simulink model "cc"  (R2015b)
settings: Solver=VariableStepAuto  StartTime=0.0  StopTime=20  RelTol=1e-3
settings Model: Creator=Oscar  LastModifiedBy=Oscar
settings DebuggingCC: MaxConsecutiveZCsMsg=none

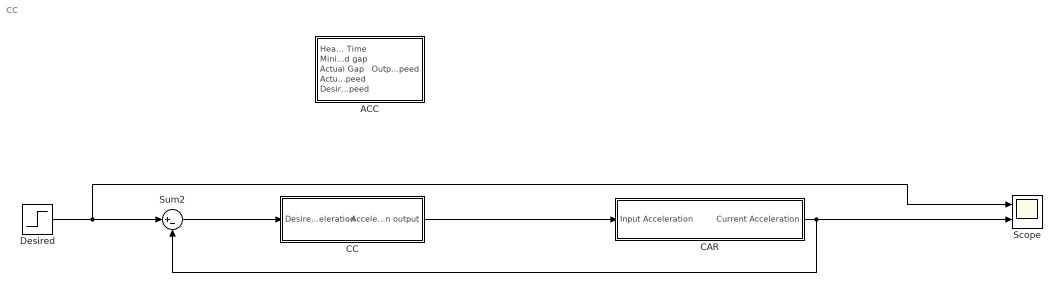
== system cc ==
  ACC : Subsystem
  "CAR " : Subsystem
  CC : Subsystem
  Desired : Step  After=1.3  SampleTime=0.0001
  Scope : Scope  NumInputPorts=2
  Sum2 : Sum  Inputs=|+-
  wires:
  Desired/1 -> Scope/1, Sum2/1
  "CAR "/1("Current Acceleration ") -> Sum2/2, Scope/2
  Sum2/1 -> CC/1(Desired Acceleration)
  CC/1(Acceleration output) -> "CAR "/1(Input Acceleration)

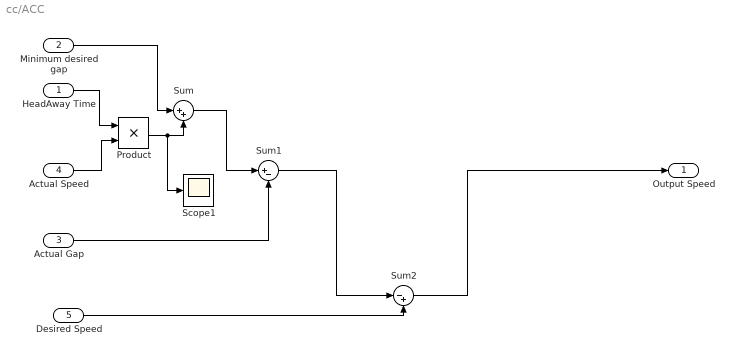
== system cc/ACC ==
  HeadAway Time : Inport
  Minimum desired gap : Inport  Port=2
  " Actual Gap" : Inport  Port=3
  " Actual Speed" : Inport  Port=4
  Desired Speed : Inport  Port=5
  Product : Product
  Scope1 : Scope
  Sum : Sum  Inputs=|++
  Sum1 : Sum  Inputs=|+-
  Sum2 : Sum  Inputs=|-+
  Output Speed : Outport
  wires:
  HeadAway Time/1 -> Product/1
  " Actual Speed"/1 -> Product/2
  Minimum desired gap/1 -> Sum/1
  Product/1 -> Scope1/1, Sum/2
  " Actual Gap"/1 -> Sum1/2
  Sum/1 -> Sum1/1
  Sum2/1 -> Output Speed/1
  Desired Speed/1 -> Sum2/2
  Sum1/1 -> Sum2/1

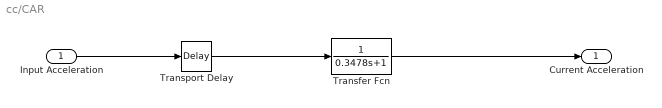
== system cc/CAR  ==
  Input Acceleration : Inport
  Transfer Fcn : TransferFcn  Denominator=[0.3478 1]
  Transport Delay : TransportDelay  DelayTime=0.4425
  "Current Acceleration " : Outport
  wires:
  Transfer Fcn/1 -> "Current Acceleration "/1
  Input Acceleration/1 -> Transport Delay/1
  Transport Delay/1 -> Transfer Fcn/1

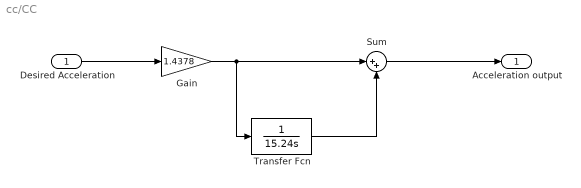
== system cc/CC ==
  Desired Acceleration : Inport
  Gain : Gain  Gain=1.4378
  Sum : Sum  Inputs=|++
  Transfer Fcn : TransferFcn  Denominator=[15.24 0]
  Acceleration output : Outport
  wires:
  Desired Acceleration/1 -> Gain/1
  Gain/1 -> Transfer Fcn/1, Sum/1
  Transfer Fcn/1 -> Sum/2
  Sum/1 -> Acceleration output/1
